simulink model "fuelcell2"  (R2021a)
settings: Solver=VariableStepAuto  StartTime=0.0  StopTime=5  RelTol=1e-3
libraries: spsSeriesRLCBranchLib x5, spsIGBTLib x3, spsVoltageMeasurementLib x2, spspowerguiLib x2, spsDiodeLib x2, spsFuelCellStackLib x1
settings Model: Creator=Dell  LastModifiedBy=Dell

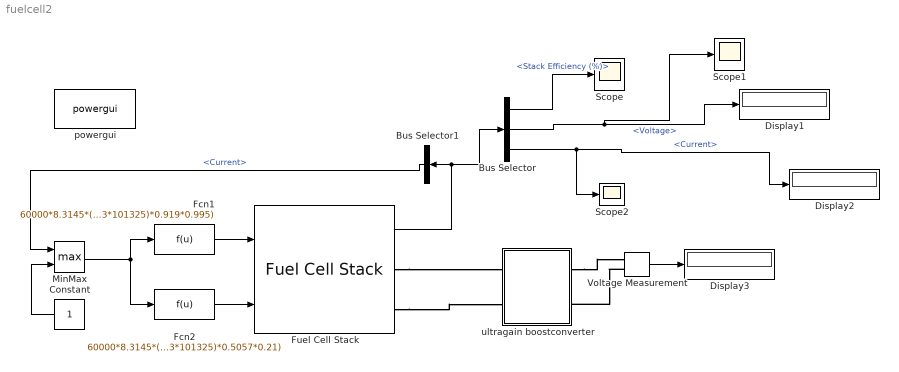
== system fuelcell2 ==
  Bus Selector : BusSelector  OutputSignals=Stack Efficiency (%),Voltage,Current
  Bus Selector1 : BusSelector  OutputSignals=Current
  Constant : Constant
  Display1 : Display
  Display2 : Display
  Display3 : Display
  Fcn1 : Fcn  Expr=60000*8.3145*(273+95)*400*u(1)/(2*96485*(3*101325)*0.919*0.995)
  Fcn2 : Fcn  Expr=60000*8.3145*(273+95)*400*u(1)/(4*96485*(3*101325)*0.5057*0.21)
  Fuel Cell Stack : spsFuelCellStackLib/Fuel Cell Stack  PresetModel=PEMFC - 1.26 kW - 24 Vdc  FcType=0  Detailed=Detailed  Eoc=[42,35]  NomVI=[52,24.23]  EndVI=[100,20]  Nc=42  n=46  TOp=55  AirFr=2400  SuppPress=[1.5,1]  Comp=[99.95,21,1]  SignX=off  SignY=off  FlowRateH2=on  FlowRateAir=on  SystemTemp=off  SystemPH2=off  SystemPAir=off  FCDyn=off  FC_tau=1  Peak_O2=80  V_Under=10
      settings: SourceProductBaseCode=PS
  MinMax : MinMax  Function=max  Inputs=2
  Scope : Scope
  Scope1 : Scope
  Scope2 : Scope
  Voltage Measurement : spsVoltageMeasurementLib/Voltage Measurement  PhasorSimulation=off  OutputType=Complex  PSBequivalent=0
  powergui : spspowerguiLib/powergui  Priority=1  SimulationMode=Discrete  SampleTime=5e-05  frequency=60  Iterations=50  frequencyindice=0  Pbase=100e6  ErrMax=1e-4  UnitsV=kV  UnitsW=MW  buscounter=0  FunctionMessages=off  echomessages=off  EnableUseOfTLC=off  CurrentSourceSwitches=off  DisableSnubberDevices=off  DisableRonSwitches=off  DisableVfSwitches=off  DisplayEquations=off  AutomaticDiscreteSolvers=off  SolverType=Tustin/Backward Euler (TBE)  Interpol=off  ExternalGateDelay=off  methode=off  Ts=100  x0status=blocks  SPID=on  SwTol=0  HookPort=off  NonlinearTolerance=1e-4  nMaxIteration=100  ContinueOnMaxIteration=off  RestoreLinks=warning  ResistiveCurrentMeasurement=off  Frange=[0:2:500]  Ylog=off  Xlog=on  ShowGrid=off  save=off  variable=ZData  structure=0  ZoomFFT=off  StartTime=0.0  cycles=1  DisplayStyle=1  fundamental=60  FreqAxis=off  MaxFrequency=1000  frequencyindicesteady=1  RmsSteady=1  display=off
  ultragain boostconverter : Subsystem
  wires:
  Fcn1/1 -> Fuel Cell Stack/1
  Bus Selector1/1 -> MinMax/1  "<Current>"
  Fcn2/1 -> Fuel Cell Stack/2
  Bus Selector/1 -> Scope/1  "<Stack Efficiency (%)>"
  Bus Selector/3 -> Display2/1, Scope2/1  "<Current>"
  Fuel Cell Stack/1 -> Bus Selector/1, Bus Selector1/1
  Bus Selector/2 -> Display1/1, Scope1/1  "<Voltage>"
  Constant/1 -> MinMax/2
  MinMax/1 -> Fcn1/1, Fcn2/1
  Voltage Measurement/1 -> Display3/1
  connections:
  Fuel Cell Stack/RConn1 -- ultragain boostconverter/LConn1
  Fuel Cell Stack/RConn2 -- ultragain boostconverter/LConn2
  ultragain boostconverter/RConn1 -- Voltage Measurement/LConn1
  Voltage Measurement/LConn2 -- ultragain boostconverter/RConn2

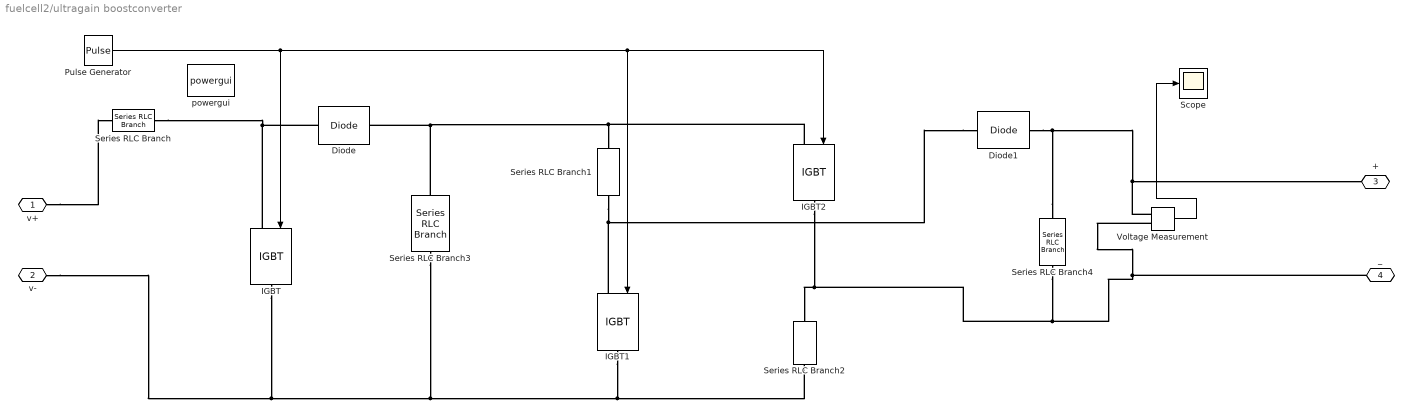
== system fuelcell2/ultragain boostconverter ==
  Diode : spsDiodeLib/Diode  Ron=0.01  Lon=0  Vf=0.3  IC=0  UseSnubber=off  Rs=50000  Cs=250e-9  Measurements=off
  Diode1 : spsDiodeLib/Diode  Ron=0.01  Lon=0  Vf=0.3  IC=0  UseSnubber=off  Rs=50000  Cs=250e-9  Measurements=off
  IGBT : spsIGBTLib/IGBT  Ron=0.001  Lon=0  Vf=1  Tf=1e-6  Tt=2e-6  IC=0  Rs=1e5  Cs=inf  Measurements=off
  IGBT1 : spsIGBTLib/IGBT  Ron=0.001  Lon=0  Vf=1  Tf=1e-6  Tt=2e-6  IC=0  Rs=1e5  Cs=inf  Measurements=off
  IGBT2 : spsIGBTLib/IGBT  Ron=0.001  Lon=0  Vf=1  Tf=1e-6  Tt=2e-6  IC=0  Rs=1e5  Cs=inf  Measurements=off
  Pulse Generator : DiscretePulseGenerator  PulseType=Time based  Period=1/30000  PulseWidth=35
  Scope : Scope
  Series RLC Branch : spsSeriesRLCBranchLib/Series RLC Branch  LConnTagsString=__new0  RConnTagsString=__new0  BranchType=L  Resistance=1  Inductance=3e-3  SetiL0=off  InitialCurrent=0  Capacitance=1e-6  Setx0=off  InitialVoltage=0  Measurements=None
  Series RLC Branch1 : spsSeriesRLCBranchLib/Series RLC Branch  LConnTagsString=__new0  RConnTagsString=__new0  BranchType=L  Resistance=1  Inductance=3e-3  SetiL0=off  InitialCurrent=0  Capacitance=1e-6  Setx0=off  InitialVoltage=0  Measurements=None
  Series RLC Branch2 : spsSeriesRLCBranchLib/Series RLC Branch  LConnTagsString=__new0  RConnTagsString=__new0  BranchType=L  Resistance=1  Inductance=3e-3  SetiL0=off  InitialCurrent=0  Capacitance=1e-6  Setx0=off  InitialVoltage=0  Measurements=None
  Series RLC Branch3 : spsSeriesRLCBranchLib/Series RLC Branch  LConnTagsString=__new0  RConnTagsString=__new0  BranchType=C  Resistance=1  Inductance=1e-3  SetiL0=off  InitialCurrent=0  Capacitance=260e-6  Setx0=off  InitialVoltage=0  Measurements=None
  Series RLC Branch4 : spsSeriesRLCBranchLib/Series RLC Branch  LConnTagsString=__new0  RConnTagsString=__new0  BranchType=C  Resistance=1  Inductance=1e-3  SetiL0=off  InitialCurrent=0  Capacitance=260e-6  Setx0=off  InitialVoltage=0  Measurements=None
  Voltage Measurement : spsVoltageMeasurementLib/Voltage Measurement  PhasorSimulation=off  OutputType=Complex  PSBequivalent=0
  powergui : spspowerguiLib/powergui  Priority=1  SimulationMode=Continuous  SampleTime=1e-5  frequency=60  Iterations=50  frequencyindice=0  Pbase=100e6  ErrMax=1e-4  UnitsV=kV  UnitsW=MW  buscounter=0  FunctionMessages=off  echomessages=off  EnableUseOfTLC=off  CurrentSourceSwitches=off  DisableSnubberDevices=off  DisableRonSwitches=off  DisableVfSwitches=off  DisplayEquations=off  AutomaticDiscreteSolvers=off  SolverType=Tustin/Backward Euler (TBE)  Interpol=off  ExternalGateDelay=off  methode=off  Ts=100  x0status=blocks  SPID=on  SwTol=0  HookPort=off  NonlinearTolerance=1e-4  nMaxIteration=100  ContinueOnMaxIteration=off  RestoreLinks=warning  ResistiveCurrentMeasurement=off  Frange=[0:2:500]  Ylog=off  Xlog=on  ShowGrid=off  save=off  variable=ZData  structure=0  ZoomFFT=off  StartTime=0.0  cycles=1  DisplayStyle=1  fundamental=60  FreqAxis=off  MaxFrequency=1000  frequencyindicesteady=1  RmsSteady=1  display=off
  v+ : PMIOPort  Side=Left
  v- : PMIOPort  Port=2  Side=Left
  + : PMIOPort  Port=3  Side=Right
  _ : PMIOPort  Port=4  Side=Right
  wires:
  Pulse Generator/1 -> IGBT/1, IGBT2/1, IGBT1/1
  Voltage Measurement/1 -> Scope/1
  connections:
  v+/RConn1 -- Series RLC Branch/LConn1
  Series RLC Branch/RConn1 -- IGBT/LConn1 -- Diode/LConn1
  Diode1/LConn1 -- IGBT1/LConn1 -- Series RLC Branch1/RConn1
  Series RLC Branch4/LConn1 -- Diode1/RConn1 -- +/RConn1 -- Voltage Measurement/LConn1
  Voltage Measurement/LConn2 -- _/RConn1 -- Series RLC Branch4/RConn1 -- IGBT2/RConn1 -- Series RLC Branch2/LConn1
  Series RLC Branch3/LConn1 -- Diode/RConn1 -- IGBT2/LConn1 -- Series RLC Branch1/LConn1
  Series RLC Branch2/RConn1 -- IGBT1/RConn1 -- IGBT/RConn1 -- v-/RConn1 -- Series RLC Branch3/RConn1
